simulink model "Simulink_3"  (R2013b)
settings: Solver=ode45  StartTime=0.0  StopTime=100.0  RelTol=1e-5
settings Model: Creator=99900361  LastModifiedBy=99900361
settings DataIOCC: SignalLoggingSaveFormat=ModelDataLogs  SignalLoggingName=sigsOut
settings DebuggingCC: SaveWithParameterizedLinksMsg=none  SignalResolutionControl=TryResolveAllWithWarning  SolverPrmCheckMsg=none  MultiTaskDSMMsg=warning  MultiTaskCondExecSysMsg=none  StrictBusMsg=None
settings HardwareCC: TargetUnknown=on
settings RTWCC: IncludeERTFirstTime=on
settings GRTTargetCC: CombineOutputUpdateFcns=off  GRTInterface=on

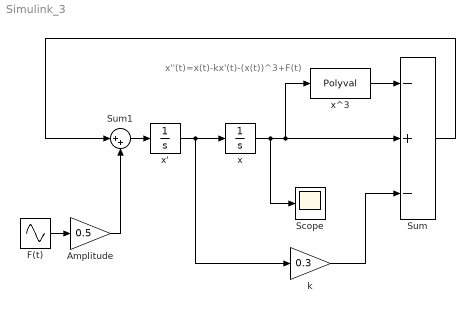
== system Simulink_3 ==
  note: x''(t)=x(t)-kx'(t)-(x(t))^3+F(t)
  Amplitude : Gain  Gain=0.5  SaturateOnIntegerOverflow=on  OutDataTypeStr=Inherit: Same as input  ParamDataTypeStr=Inherit: Same as input
  F(t) : Sin  Frequency=1.25  Phase=pi/2  SampleTime=0
  Scope : Scope
  Sum : Sum  Inputs=-+-  SaturateOnIntegerOverflow=on
  Sum1 : Sum  Inputs=|++  SaturateOnIntegerOverflow=on
  k : Gain  Gain=0.3  SaturateOnIntegerOverflow=on  OutDataTypeStr=Inherit: Same as input  ParamDataTypeStr=Inherit: Same as input
  x : Integrator  InitialCondition=1
  x' : Integrator  InitialCondition=1
  x^3 : Polyval  Coefs=[1,0,0,0]
  wires:
  x'/1 -> x/1, k/1
  x/1 -> Scope/1, Sum/2, x^3/1
  Sum1/1 -> x'/1
  k/1 -> Sum/3
  Sum/1 -> Sum1/1
  x^3/1 -> Sum/1
  F(t)/1 -> Amplitude/1
  Amplitude/1 -> Sum1/2
